simulink model "nonlinear_control"  (R2024b)
settings: Solver=VariableStepAuto  StartTime=0.0  StopTime=20.0  FixedStep=0.04  RelTol=1e-6  AbsTol=1e-8
undefined symbols (not defined in the file): Kd_theta, Kp_theta, params, x0
settings Model: Creator=Pinoi  LastModifiedBy=david

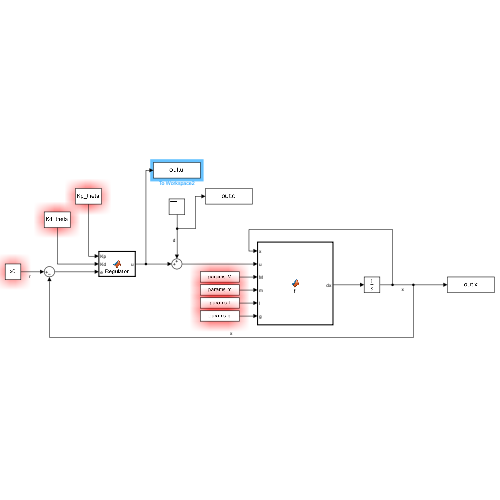
[thumbnail: Simulink's stored preview of the top-level diagram]
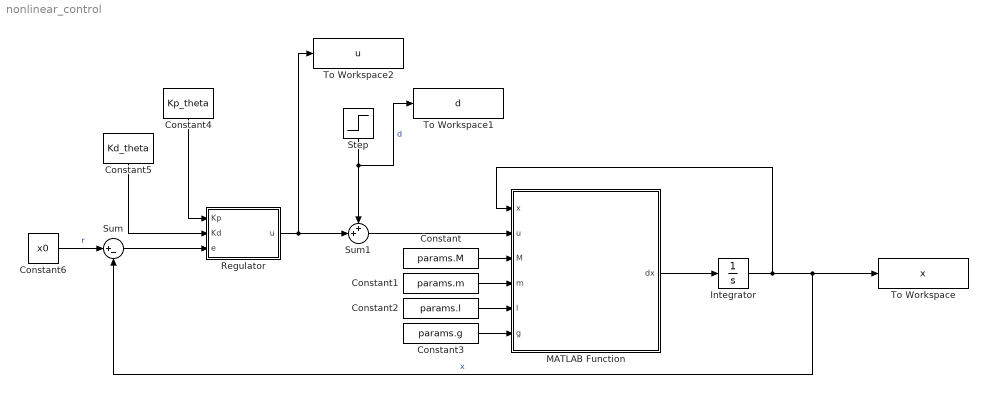
== system nonlinear_control ==
  Constant : Constant  Value=params.M
  Constant1 : Constant  Value=params.m
  Constant2 : Constant  Value=params.l
  Constant3 : Constant  Value=params.g
  Constant4 : Constant  Value=Kp_theta
  Constant5 : Constant  Value=Kd_theta
  Constant6 : Constant  Value=x0
  Integrator : Integrator  InitialCondition=[0;0;0;0]
  MATLAB Function : MATLAB Function  TreatAsAtomicUnit=on
  Regulator : MATLAB Function  TreatAsAtomicUnit=on
  Step : Step  Time=0.1  Before=1  After=0  SampleTime=0
  Sum : Sum  Inputs=|+-
  Sum1 : Sum  Inputs=++|
  To Workspace : ToWorkspace  VariableName=x  SampleTime=-1
      settings: Save2DSignal=2-D array (concatenate along first dimension)
  To Workspace1 : ToWorkspace  VariableName=d  SampleTime=-1
      settings: Save2DSignal=2-D array (concatenate along first dimension)
  To Workspace2 : ToWorkspace  VariableName=u  SampleTime=-1
      settings: Save2DSignal=2-D array (concatenate along first dimension)
  wires:
  MATLAB Function/1(dx) -> Integrator/1
  Integrator/1 -> MATLAB Function/1(x), Sum/2, To Workspace/1  "x"
  Sum/1 -> Regulator/3(e)
  Constant/1 -> MATLAB Function/3(M)
  Constant2/1 -> MATLAB Function/5(l)
  Constant3/1 -> MATLAB Function/6(g)
  Regulator/1(u) -> Sum1/2, To Workspace2/1
  Sum1/1 -> MATLAB Function/2(u)
  Step/1 -> To Workspace1/1, Sum1/1  "d"
  Constant6/1 -> Sum/1  "r"
  Constant1/1 -> MATLAB Function/4(m)
  Constant4/1 -> Regulator/1(Kp)
  Constant5/1 -> Regulator/2(Kd)

== matlab function nonlinear_control/Regulator ==
  data: Kp input; Kd input; e input; u output
function u = Regulator(Kp,Kd,e)

pd = @(x) Kp * e(3) + Kd * e(4);
u=pd(e);

== matlab function nonlinear_control/MATLAB Function ==
  data: x input; u input; dx output; M input; m input; l input; g input
function dx = f( x, u, M, m, l, g)

 dx=[
     x(2); % dx
     (m*l*x(4)^2*sin(x(3))+m*g*sin(x(3))*cos(x(3))+u)/(M+m*sin(x(3))^2); % d2x
     x(4);  % dtheta
     ((M+m)*g/l*sin(x(3))-m*x(4)^2*cos(x(3))*sin(x(3))+(u)*cos(x(3))/l)/...
     (M+m*sin(x(3))^2)]; %d2theta

end
